simulink model "fh_system"  (Simulink 7.2)
settings: Solver=ode23  StartTime=0.0  StopTime=0.2  RelTol=1e-3
undefined symbols (not defined in the file or in its folder): sigbuilder_block
libraries: dsparch4 x5, commsynccomp2 x2, dspbuff3 x2, simulink x1, dspsigattribs x1, commutil2 x1, commseqgen2 x1, commfilt2 x1
settings Model: Creator=Administrator  LastModifiedBy=Administrator
settings OptimizationCC: InitFltsAndDblsToZero=on
settings DebuggingCC: SaveWithParameterizedLinksMsg=none  SignalResolutionControl=TryResolveAllWithWarning  MultiTaskDSMMsg=warning  MultiTaskCondExecSysMsg=none
settings RTWCC: IncludeERTFirstTime=on
settings GRTTargetCC: TargetFcnLib=ansi_tfl_tmw.mat

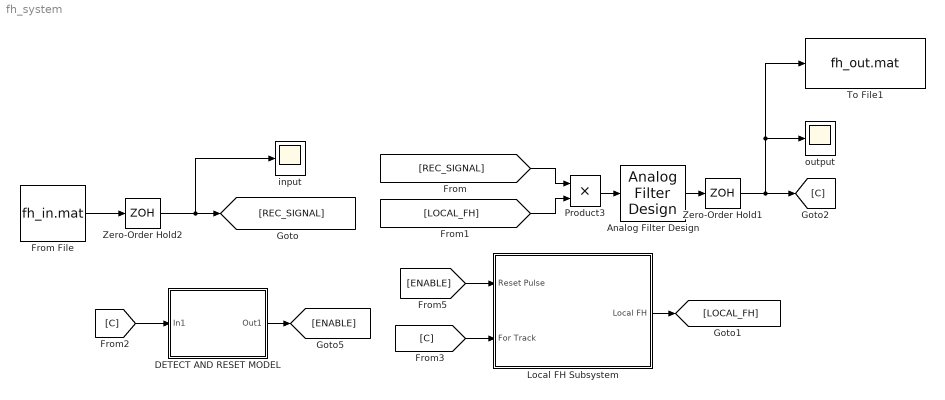
== system fh_system ==
  Analog Filter Design : dsparch4/Analog Filter Design  method=Butterworth  filttype=Bandpass  N=8  Wlo=1900*pi  Whi=2100*pi  Rp=2  Rs=40
  DETECT AND RESET MODEL : Subsystem
  From File : FromFile  FileName=fh_in.mat  SampleTime=1/700000
  Local FH Subsystem : Subsystem
  Product3 : Product  OutDataType=sfix(16)  OutScaling=2^0  RndMeth=Zero
  To File1 : ToFile  Filename=fh_out.mat  MatrixName=fh_out
  Zero-Order Hold1 : ZeroOrderHold  SampleTime=1/700000
  Zero-Order Hold2 : ZeroOrderHold  SampleTime=1/700000
  input : Scope
      settings: YMin=-0.55  YMax=0.55  SaveName=ScopeData2
  output : Scope
      settings: YMin=-0.55  YMax=0.55
  wires:
  From File/1 -> Zero-Order Hold2/1
  Local FH Subsystem/1(Local FH) -> [LOCAL_FH]
  [C] -> DETECT AND RESET MODEL/1(In1)
  [ENABLE] -> Local FH Subsystem/1(Reset Pulse)
  DETECT AND RESET MODEL/1(Out1) -> [ENABLE]
  Analog Filter Design/1 -> Zero-Order Hold1/1
  [REC_SIGNAL] -> Product3/1
  [LOCAL_FH] -> Product3/2
  Product3/1 -> Analog Filter Design/1
  [C] -> Local FH Subsystem/2(For Track)
  Zero-Order Hold2/1 -> [REC_SIGNAL], input/1
  Zero-Order Hold1/1 -> [C], output/1, To File1/1

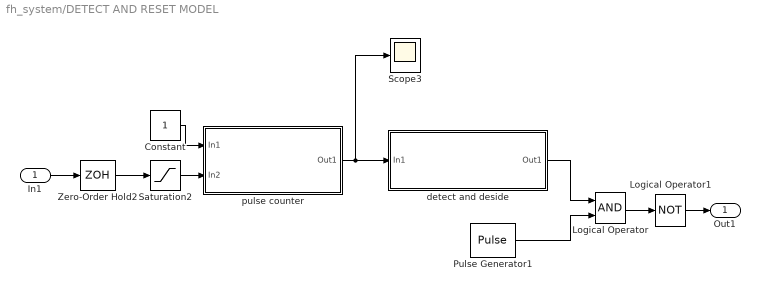
== system fh_system/DETECT AND RESET MODEL ==
  In1 : Inport  OutDataType=sfix(16)  OutScaling=2^0
  Constant : Constant  OutDataType=sfix(16)  OutScaling=2^0
  Logical Operator : Logic  AllPortsSameDT=off  OutDataTypeMode=boolean  OutDataTypeStr=boolean
  Logical Operator1 : Logic  Operator=NOT  AllPortsSameDT=off  OutDataTypeMode=boolean  OutDataTypeStr=boolean
  Pulse Generator1 : DiscretePulseGenerator  PulseType=Time based  Period=0.02  PulseWidth=50
  Saturation2 : Saturate  SampleTime=0.0001
  Scope3 : Scope
      settings: YMin=-0.275  YMax=0.275  SaveName=ScopeData27
  Zero-Order Hold2 : ZeroOrderHold  SampleTime=1/700000
  detect and deside : Subsystem
  pulse counter : Subsystem
  Out1 : Outport  OutDataType=sfix(16)  OutScaling=2^0
  wires:
  Constant/1 -> pulse counter/1(In1)
  detect and deside/1(Out1) -> Logical Operator/1
  pulse counter/1(Out1) -> detect and deside/1(In1), Scope3/1
  Logical Operator/1 -> Logical Operator1/1
  Pulse Generator1/1 -> Logical Operator/2
  Saturation2/1 -> pulse counter/2(In2)
  In1/1 -> Zero-Order Hold2/1
  Logical Operator1/1 -> Out1/1
  Zero-Order Hold2/1 -> Saturation2/1

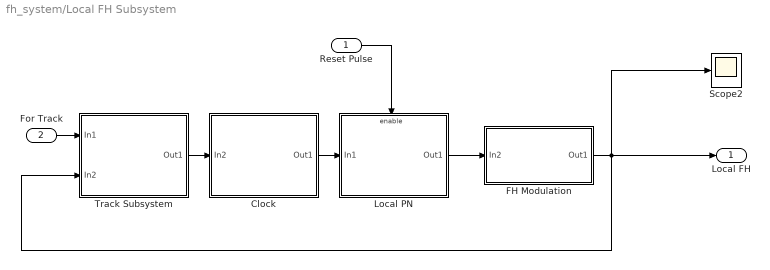
== system fh_system/Local FH Subsystem ==
  Reset Pulse : Inport  OutDataType=sfix(16)  OutScaling=2^0
  For Track : Inport  Port=2  OutDataType=sfix(16)  OutScaling=2^0
  Clock : Subsystem  TreatAsAtomicUnit=on
  FH Modulation : Subsystem
  Local PN : Subsystem  TreatAsAtomicUnit=on
  Scope2 : Scope
      settings: YMin=-2  YMax=2  SaveName=ScopeData9
  Track Subsystem : Subsystem  TreatAsAtomicUnit=on
  Local FH : Outport  OutDataType=sfix(16)  OutScaling=2^0
  wires:
  Local PN/1(Out1) -> FH Modulation/1(In2)
  FH Modulation/1(Out1) -> Scope2/1, Track Subsystem/2(In2), Local FH/1
  Clock/1(Out1) -> Local PN/1(In1)
  Reset Pulse/1 -> Local PN/Enable
  Track Subsystem/1(Out1) -> Clock/1(In2)
  For Track/1 -> Track Subsystem/1(In1)

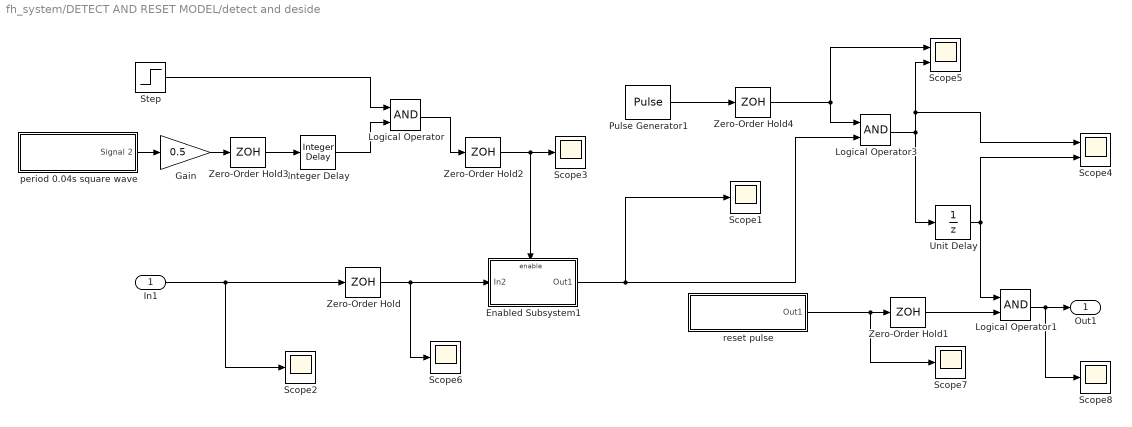
== system fh_system/DETECT AND RESET MODEL/detect and deside ==
  In1 : Inport  OutDataType=sfix(16)  OutScaling=2^0
  Enabled Subsystem1 : Subsystem  TreatAsAtomicUnit=on
  Gain : Gain  Gain=0.5  ParameterDataType=sfix(16)  ParameterScaling=2^0  OutDataType=sfix(16)  OutScaling=2^0
  Integer Delay : simulink/Discrete/Integer Delay  vinit=0.0  samptime=-1  NumDelays=2
  Logical Operator : Logic  AllPortsSameDT=off  OutDataTypeMode=boolean  OutDataTypeStr=boolean
  Logical Operator1 : Logic  AllPortsSameDT=off  OutDataTypeMode=boolean  OutDataTypeStr=boolean
  Logical Operator3 : Logic  AllPortsSameDT=off  OutDataTypeMode=boolean  OutDataTypeStr=boolean
  Pulse Generator1 : DiscretePulseGenerator  PulseType=Time based  Period=0.04  PulseWidth=50  PhaseDelay=0.02
  Scope{1..3,6..8} (6 alike) : Scope
      Scope1 settings: YMin=0.95  YMax=1.05  SaveName=ScopeData20
      Scope2 settings: YMin=-1  YMax=1  SaveName=ScopeData21
      Scope3 settings: YMin=0  YMax=1  SaveName=ScopeData24
      Scope6 settings: YMin=-1  YMax=1  SaveName=ScopeData23
      Scope7 settings: YMin=0  YMax=1  SaveName=ScopeData7
      Scope8 settings: YMin=0  YMax=1  SaveName=ScopeData14
  Scope4 : Scope  NumInputPorts=2
      settings: TimeRange=0.2  YMin=0~0  YMax=1~1  SaveName=ScopeData11
  Scope5 : Scope  NumInputPorts=2
      settings: YMin=0~0  YMax=1~1  SaveName=ScopeData16
  Step : Step  Time=0.04  SampleTime=0
  Unit Delay : UnitDelay  SampleTime=0.01
  Zero-Order Hold : ZeroOrderHold  SampleTime=0.001
  Zero-Order Hold{1..4} (4 alike) : ZeroOrderHold  SampleTime=0.01
  period 0.04s square wave : Subsystem  Tag=STV Subsys  LoadFcn=sigbuilder_block('load');  StartFcn=sigbuilder_block('start');  StopFcn=sigbuilder_block('stop');  ClipboardFcn=sigbuilder_block('clipboard');  mask(Sigbuilder block){}
      mask help: Sigbuilder GUI
      mask init:
      | if ~strcmp(get_param(bdroot(gcbh),'SimulationStatus'),'stopped') tuvar = sigbuilder_block('maskInit'); end
      settings: CopyFcn=sigbuilder_block('copy');  DeleteFcn=sigbuilder_block('delete');  ModelCloseFcn=sigbuilder_block('modelClose');  PreSaveFcn=sigbuilder_block('preSave');  NameChangeFcn=sigbuilder_block('namechange');  OpenFcn=sigbuilder_block('open',[3 19.5 762 498 ]);  CloseFcn=sigbuilder_block('close');
      mask Display: plot(0,0,100,100,[10,10,40,40,10],[80,20,20,80,80],[40,10],[50,50], [40,27,10],[65,72,56],[40,25,25,10],[28,28,43,43]);
  reset pulse : Subsystem
  Out1 : Outport  OutDataType=sfix(16)  OutScaling=2^0
  wires:
  In1/1 -> Zero-Order Hold/1, Scope2/1
  Enabled Subsystem1/1(Out1) -> Scope1/1, Logical Operator3/2
  Zero-Order Hold/1 -> Enabled Subsystem1/1(In2), Scope6/1
  Zero-Order Hold2/1 -> Scope3/1, Enabled Subsystem1/Enable
  Step/1 -> Logical Operator/1
  period 0.04s square wave/1(Signal 2) -> Gain/1
  Logical Operator/1 -> Zero-Order Hold2/1
  Gain/1 -> Zero-Order Hold3/1
  Zero-Order Hold3/1 -> Integer Delay/1
  Integer Delay/1 -> Logical Operator/2
  Pulse Generator1/1 -> Zero-Order Hold4/1
  Logical Operator3/1 -> Unit Delay/1, Scope5/2, Scope4/1
  Zero-Order Hold4/1 -> Logical Operator3/1, Scope5/1
  Logical Operator1/1 -> Out1/1, Scope8/1
  Unit Delay/1 -> Logical Operator1/1, Scope4/2
  reset pulse/1(Out1) -> Scope7/1, Zero-Order Hold1/1
  Zero-Order Hold1/1 -> Logical Operator1/2

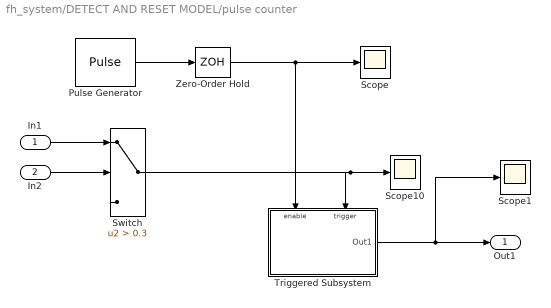
== system fh_system/DETECT AND RESET MODEL/pulse counter ==
  In1 : Inport  OutDataType=sfix(16)  OutScaling=2^0
  In2 : Inport  Port=2  OutDataType=sfix(16)  OutScaling=2^0
  Pulse Generator : DiscretePulseGenerator  PulseType=Time based  Period=0.04  PulseWidth=50  PhaseDelay=0.01
  Scope : Scope
      settings: YMin=0  YMax=1  SaveName=ScopeData28
  Scope1 : Scope
      settings: YMin=5  YMax=11  SaveName=ScopeData8
  Scope10 : Scope
      settings: YMin=-2  YMax=2  SaveName=ScopeData10
  Switch : Switch  Criteria=u2 > Threshold  Threshold=0.3
  Triggered Subsystem : Subsystem  TreatAsAtomicUnit=on
  Zero-Order Hold : ZeroOrderHold  SampleTime=0.01
  Out1 : Outport  OutDataType=sfix(16)  OutScaling=2^0
  wires:
  In2/1 -> Switch/2
  Pulse Generator/1 -> Zero-Order Hold/1
  Zero-Order Hold/1 -> Scope/1, Triggered Subsystem/Enable
  In1/1 -> Switch/1
  Switch/1 -> Triggered Subsystem/Trigger, Scope10/1
  Triggered Subsystem/1(Out1) -> Out1/1, Scope1/1

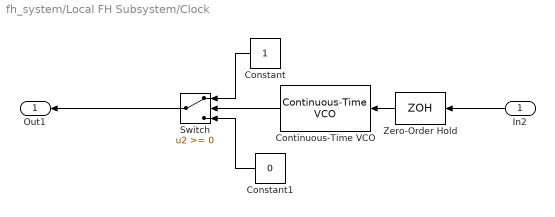
== system fh_system/Local FH Subsystem/Clock ==
  In2 : Inport  Orientation=left  OutDataType=sfix(16)  OutScaling=2^0
  Constant : Constant  Orientation=left  OutDataType=sfix(16)  OutScaling=2^0
  Constant1 : Constant  Orientation=left  Value=0  OutDataType=sfix(16)  OutScaling=2^0
  Continuous-Time VCO : commsynccomp2/Continuous-Time VCO  Orientation=left  SystemSampleTime=-1  Ac=1  Fc=100  Kc=0.1  Ph=-pi/2
  Switch : Switch  Orientation=left
  Zero-Order Hold : ZeroOrderHold  Orientation=left  SampleTime=1000
  Out1 : Outport  Orientation=left  OutDataType=sfix(16)  OutScaling=2^0
  wires:
  Constant1/1 -> Switch/3
  Constant/1 -> Switch/1
  Continuous-Time VCO/1 -> Switch/2
  Switch/1 -> Out1/1
  In2/1 -> Zero-Order Hold/1
  Zero-Order Hold/1 -> Continuous-Time VCO/1

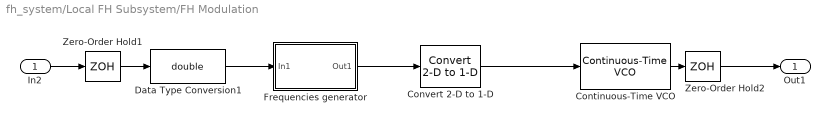
== system fh_system/Local FH Subsystem/FH Modulation ==
  In2 : Inport
  Continuous-Time VCO : commsynccomp2/Continuous-Time VCO  SystemSampleTime=-1  Ac=1  Fc=70000  Kc=1000  Ph=0
  Convert 2-D to 1-D : dspsigattribs/Convert 2-D to 1-D  SystemSampleTime=-1
  Data Type Conversion1 : DataTypeConversion  OutDataTypeMode=double  OutDataType=sfix(16)  OutScaling=2^0  OutDataTypeStr=double
  Frequencies generator : Subsystem
  Zero-Order Hold1 : ZeroOrderHold  SampleTime=0.01
  Zero-Order Hold2 : ZeroOrderHold  SampleTime=1/700000
  Out1 : Outport
  wires:
  Frequencies generator/1(Out1) -> Convert 2-D to 1-D/1
  Continuous-Time VCO/1 -> Zero-Order Hold2/1
  In2/1 -> Zero-Order Hold1/1
  Zero-Order Hold2/1 -> Out1/1
  Zero-Order Hold1/1 -> Data Type Conversion1/1
  Data Type Conversion1/1 -> Frequencies generator/1(In1)
  Convert 2-D to 1-D/1 -> Continuous-Time VCO/1

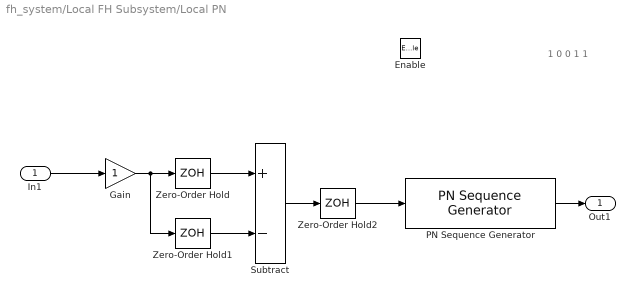
== system fh_system/Local FH Subsystem/Local PN ==
  note: 1 0 0 1 1
  In1 : Inport  OutDataType=sfix(16)  OutScaling=2^0
  Enable : EnablePort  StatesWhenEnabling=reset
  Gain : Gain  ParameterDataType=sfix(16)  ParameterScaling=2^0  OutDataType=sfix(16)  OutScaling=2^0
  PN Sequence Generator : commseqgen2/PN Sequence Generator  poly=[1 0 0 1 1]  ini_sta=[0 0 0 1]  outBitMaskSource=Dialog parameter  shift=0  Ts=0.01  frameBased=off  sampPerFrame=1  reset=on  bitPackedOutputs=off  outDataType=double  numPackedBits=8  bitPackDataSigned=off  bitPackedOutDType=double
  Subtract : Sum  Inputs=+-  OutDataType=sfix(16)  OutScaling=2^-10
  Zero-Order Hold : ZeroOrderHold
  Zero-Order Hold1 : ZeroOrderHold
  Zero-Order Hold2 : ZeroOrderHold  SampleTime=0.01
  Out1 : Outport  OutDataType=sfix(16)  OutScaling=2^0
  wires:
  PN Sequence Generator/1 -> Out1/1
  In1/1 -> Gain/1
  Gain/1 -> Zero-Order Hold/1, Zero-Order Hold1/1
  Subtract/1 -> Zero-Order Hold2/1
  Zero-Order Hold/1 -> Subtract/1
  Zero-Order Hold1/1 -> Subtract/2
  Zero-Order Hold2/1 -> PN Sequence Generator/1

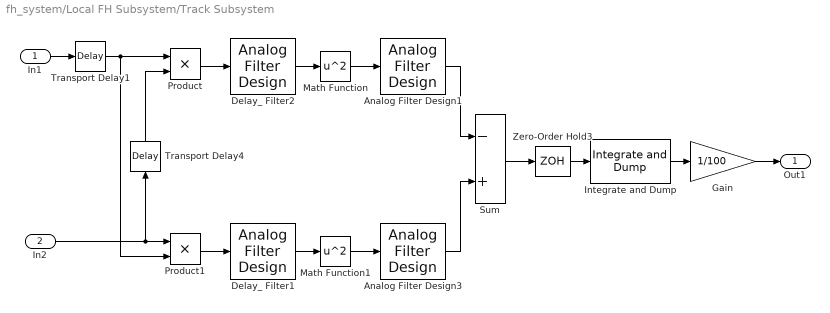
== system fh_system/Local FH Subsystem/Track Subsystem ==
  In1 : Inport  OutDataType=sfix(16)  OutScaling=2^0
  In2 : Inport  Port=2  OutDataType=sfix(16)  OutScaling=2^0
  Analog Filter Design1 : dsparch4/Analog Filter Design  method=Butterworth  filttype=Lowpass  N=8  Wlo=2000*pi  Whi=80  Rp=2  Rs=40
  Analog Filter Design3 : dsparch4/Analog Filter Design  method=Butterworth  filttype=Lowpass  N=8  Wlo=2000*pi  Whi=80  Rp=2  Rs=40
  Delay_ Filter1 : dsparch4/Analog Filter Design  method=Butterworth  filttype=Bandpass  N=8  Wlo=1900*pi  Whi=2100*pi  Rp=2  Rs=40
  Delay_ Filter2 : dsparch4/Analog Filter Design  method=Butterworth  filttype=Bandpass  N=8  Wlo=1900*pi  Whi=2100*pi  Rp=2  Rs=40
  Gain : Gain  Gain=1/100  ParameterDataType=sfix(16)  ParameterScaling=2^0  OutDataType=sfix(16)  OutScaling=2^0
  Integrate and Dump : commfilt2/Integrate and Dump  DialogController=commDDGCreate  DialogControllerArgs=DataTag2  obssamples=100  offsetsamples=0  nodump=off  roundingMode=Floor  overflowMode=off
  Math Function : Math  Operator=square  OutDataType=sfix(16)  OutScaling=2^0  SaturateOnIntegerOverflow=on
  Math Function1 : Math  Operator=square  OutDataType=sfix(16)  OutScaling=2^0  SaturateOnIntegerOverflow=on
  Product : Product  OutDataType=sfix(16)  OutScaling=2^0  RndMeth=Zero
  Product1 : Product  OutDataType=sfix(16)  OutScaling=2^0  RndMeth=Zero
  Sum : Sum  Inputs=-+  OutDataType=sfix(16)  OutScaling=2^0
  Transport Delay1 : TransportDelay  DelayTime=0.02
  Transport Delay4 : TransportDelay  Orientation=up  DelayTime=0.04
  Zero-Order Hold3 : ZeroOrderHold  SampleTime=1/10000
  Out1 : Outport  OutDataType=sfix(16)  OutScaling=2^0
  wires:
  Transport Delay1/1 -> Product1/2, Product/1
  Product/1 -> Delay_ Filter2/1
  Product1/1 -> Delay_ Filter1/1
  Sum/1 -> Zero-Order Hold3/1
  Zero-Order Hold3/1 -> Integrate and Dump/1
  In1/1 -> Transport Delay1/1
  In2/1 -> Product1/1, Transport Delay4/1
  Transport Delay4/1 -> Product/2
  Delay_ Filter2/1 -> Math Function/1
  Math Function/1 -> Analog Filter Design1/1
  Math Function1/1 -> Analog Filter Design3/1
  Analog Filter Design1/1 -> Sum/1
  Analog Filter Design3/1 -> Sum/2
  Delay_ Filter1/1 -> Math Function1/1
  Integrate and Dump/1 -> Gain/1
  Gain/1 -> Out1/1

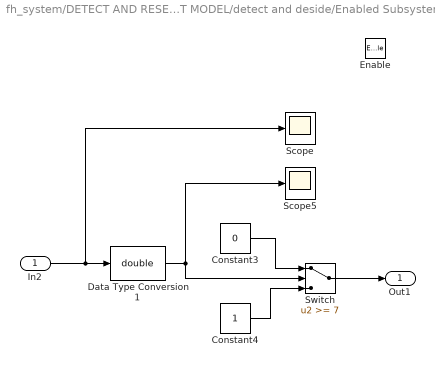
== system fh_system/DETECT AND RESET MODEL/detect and deside/Enabled Subsystem1 ==
  In2 : Inport  OutDataType=sfix(16)  OutScaling=2^0
  Enable : EnablePort  StatesWhenEnabling=reset
  Constant3 : Constant  Value=0  OutDataType=sfix(16)  OutScaling=2^0
  Constant4 : Constant  OutDataType=sfix(16)  OutScaling=2^0
  Data Type Conversion1 : DataTypeConversion  OutDataTypeMode=double  OutDataType=sfix(16)  OutScaling=2^0  OutDataTypeStr=double
  Scope : Scope
      settings: YMin=-1  YMax=1  SaveName=ScopeData12
  Scope5 : Scope
      settings: YMin=9  YMax=19  SaveName=ScopeData22
  Switch : Switch  Threshold=7
  Out1 : Outport  OutDataType=sfix(16)  OutScaling=2^0
  wires:
  In2/1 -> Scope/1, Data Type Conversion1/1
  Data Type Conversion1/1 -> Scope5/1, Switch/2
  Switch/1 -> Out1/1
  Constant4/1 -> Switch/3
  Constant3/1 -> Switch/1

== system fh_system/DETECT AND RESET MODEL/detect and deside/period 0.04s square wave ==
  Demux : Demux  Tag=STV Demux  Outputs=1
  FromWs : FromWorkspace  Tag=STV FromWs  VariableName=tuvar  SampleTime=0  SigBuilderData=DataTag0  VnvData=DataTag1
      SigBuilderData=|
      | channels.xData = [0 0.02 0.02 0.04 0.04 0.06 0.06 0.08 0.08 0.1 0.1 0.12 ... (994 elements, 1x994)]
      | channels.yData = [2 2 0 0 2 2 0 0 2 2 0 0 2 2 0 0 2 2 0 0 2 2 0 0 2 2 0 0 2 2 0 0 2 2 0 0 2 2 0 0 2 2 0 0 2 2 0 0 2 2 0 0 2 2 0 0 2 2 0 0 2 2 0 0 2 2 0 0 0 2 2 0 0 2 2 0 0 2 2 0 0 2 2 0 0 2 2 0 0 2 2 0 0 2 2 0 0 2 2 0 0 2 2 0 0 2 2 0 0 2 2 0 0 2 2 0 0 2 2 0 0 2 2 0 0 2 2 0 0 2 2 2 0 0 2 2 0 0 2 2 0 0 2 2 0 0 2 2 0 0 2 2 0 0 2 2 0 0 2 2 0 0 2 2 0 0 2 2 0 0 2 2 0 0 2 2 0 0 2 2 0 0 2 2 0 0 2 2 0 0 2 2 0 0 2 2 0 0 2 2 0 0 2 2 0 0 2 2 0 0 2 2 0 0 2 2 0 0 2 2 0 0 2 2 0 0 2 2 0 0 2 2 0 0 2 2 0 0 2 2 0 0 2 2 0 0 2 2 0 0 2 2 0 0 2 2 0 0 2 2 0 0 2 2 0 0 2 2 0 0 2 2 0 0 2 2 0 0 2 2 0 0 2 2 0 0 2 2 0 0 2 2 0 0 2 2 0 0 2 2 0 0 2 2 0 0 2 2 0 0 2 2 0 0 2 2 0 0 2 2 0 0 2 2 0 0 2 2 0 0 2 2 0 0 2 2 0 0 2 2 0 0 2 2 0 0 2 2 0 0 2 2 0 0 2 2 0 0 2 2 0 0 2 2 0 0 2 2 0 0 2 2 0 0 2 2 0 0 2 2 0 0 2 2 0 0 2 2 0 0 2 2 0 0 2 2 0 0 2 2 0 0 2 2 0 0 2 2 0 0 2 2 0 0 2 2 0 0 2 2 0 0 2 2 0 0 2 2 0 0 2 2 0 0 2 2 0 0 2 2 0 0 2 2 0 0 2 2 0 0 2 2 0 0 2 2 0 0 2 2 0 0 2 2 0 0 2 2 0 0 2 2 0 0 2 2 0 0 2 2 0 0 2 2 0 0 2 2 0 0 2 2 0 0 2 2 0 0 2 2 0 0 2 2 0 0 2 2 0 0 2 2 0 0 2 2 0 0 2 2 0 0 2 2 0 0 2 2 0 0 2 2 0 0 2 2 0 0 2 2 0 0 2 2 0 0 2 2 0 0 2 2 0 0 2 2 0 0 2 2 0 0 2 2 0 0 2 2 0 0 2 2 0 0 2 2 0 0 2 2 0 0 2 2 0 0 2 2 0 0 2 2 0 0 2 2 0 0 2 2 0 0 2 2 0 0 2 2 0 0 2 2 0 0 2 2 0 0 2 2 0 0 2 2 0 0 2 2 0 0 2 2 0 0 2 2 0 0 2 2 0 0 2 2 0 0 2 2 0 0 2 2 0 0 2 2 0 0 2 2 0 0 2 2 0 0 2 2 0 0 2 2 0 0 2 2 0 0 2 2 0 0 2 2 0 0 2 2 0 0 2 2 0 0 2 2 0 0 2 2 0 0 2 2 0 0 2 2 0 0 2 2 0 0 2 2 0 0 2 2 0 0 2 2 0 0 2 2 0 0 2 2 0 0 2 2 0 0 2 2 0 0 2 2 0 0 2 2 0 0 2 2 0 0 2 2 0 0 2 2 0 0 2 2 0 0 2 2 0 0 2 2 0 0 2 2 0 0 2 2 0 0 2 2 0 0 2 2 0 0 2 2 0 0 2 2 0 0 2 2 0 0 2 2 0 0 2 2 0 0 2 2 0 0 2 2 0 0 2 2 0 0 2 2 0 0 2 2 0 0 2 2 0 0 2 2 0 0 2 2 0 0 2 2 0 0 2 2 0 0 2 2 0 0 2 2 0 0 2 2 0 0 2 2 0 0 2 2 0 0 2 2 0 0 2 2 0 0 2 2 0 0 2 2 0 0 2 2 0 0 2 2 0 0 2 2 0 0 2 2 0 0 2 2 0 0 2 2 0 0 2 2 0 0 2 2 0 0 2 2 0 0 2 2 0 0 2 2 0 0 2 2 0 0 2 2 0 0 2 2 0 0 2 2 0 0 2 2 0 0 2 2 0 0 2 2 0 0 2 2 0 0 2 2 0 0 2 2 0 0 2 2 0 0 2 2 0 0 2 2 0 0 2 2 0 0 2 2 0 0 2 2 0 0]
      | channels.label = 'Signal 2'
      | common.afterFinalStr = 'Extrapolate'
      | common.sampleTime = 0
      | dataSet.timeRange = [0 10]
      | dataSet.name = 'Group 1'
  Signal 2 : Outport  Tag=STV Outport
  wires:
  FromWs/1 -> Demux/1
  Demux/1 -> Signal 2/1

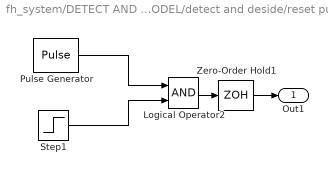
== system fh_system/DETECT AND RESET MODEL/detect and deside/reset pulse ==
  Logical Operator2 : Logic  AllPortsSameDT=off  OutDataTypeMode=boolean  OutDataTypeStr=boolean
  Pulse Generator : DiscretePulseGenerator  PulseType=Time based  Period=0.04  PulseWidth=1/4
  Step1 : Step  Time=0.08
  Zero-Order Hold1 : ZeroOrderHold  SampleTime=0.01
  Out1 : Outport  OutDataType=sfix(16)  OutScaling=2^0
  wires:
  Pulse Generator/1 -> Logical Operator2/1
  Logical Operator2/1 -> Zero-Order Hold1/1
  Step1/1 -> Logical Operator2/2
  Zero-Order Hold1/1 -> Out1/1

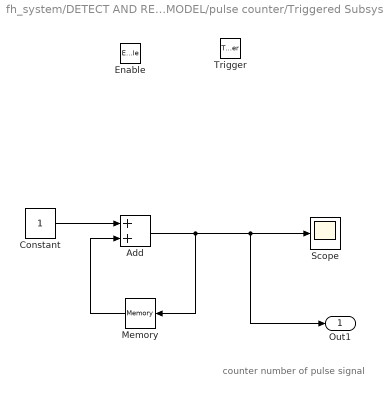
== system fh_system/DETECT AND RESET MODEL/pulse counter/Triggered Subsystem ==
  note: counter number of pulse signal
  Enable : EnablePort  StatesWhenEnabling=reset
  Trigger : TriggerPort
  Add : Sum  OutDataType=sfix(16)  OutScaling=2^-10
  Constant : Constant  OutDataType=sfix(16)  OutScaling=2^0
  Memory : Memory  Orientation=left  X0=1  InheritSampleTime=on
  Scope : Scope
      settings: TimeRange=0.03745829214038558  YMin=4.549583445310418  YMax=50.59688255845205  SaveName=ScopeData6
  Out1 : Outport  OutDataType=sfix(16)  OutScaling=2^0
  wires:
  Constant/1 -> Add/1
  Add/1 -> Memory/1, Scope/1, Out1/1
  Memory/1 -> Add/2

== system fh_system/Local FH Subsystem/FH Modulation/Frequencies generator ==
  In1 : Inport
  Bit to Integer Converter : commutil2/Bit to Integer Converter  nbits=4  bitOrder=MSB first  signedOutputValues=Unsigned  outDtype=Same as input  outDtypeSigned=Inherit via internal rule
  Buffer : dspbuff3/Buffer  N=4  V=3  ic=0
  Unbuffer : dspbuff3/Unbuffer  ic=4
  Out1 : Outport
  wires:
  Buffer/1 -> Bit to Integer Converter/1
  Bit to Integer Converter/1 -> Unbuffer/1
  In1/1 -> Buffer/1
  Unbuffer/1 -> Out1/1
